simulink model "ES101A_DiagcMgr"  (R2013b)
settings: Solver=ode45  StartTime=0.0  StopTime=0.44  RelTol=1e-3
values from neighbouring files (symbols this model uses):
  BrdgVltg = DataDict.IpSignal    [ES101A_DiagcMgr_DataDict.m]
  DEM_CLEAR_PENDING = DataDict.Constant    [ES101A_DiagcMgr_DataDict.m]
  DEM_DTC_GROUP_ALL_DTCS = DataDict.Constant    [ES101A_DiagcMgr_DataDict.m]
  DFTAGICNTR_CNT_U08 = DataDict.Constant    [ES101A_DiagcMgr_DataDict.m]
  DIAGCMGR_NTCINFOSTSTESTFAILD_CNT_U08 = DataDict.Constant    [ES101A_DiagcMgr_DataDict.m]
  DIAGCMGR_NTCINFOSTSTESTFAILDTHISIGNCYC_CNT_U08 = DataDict.Constant    [ES101A_DiagcMgr_DataDict.m]
  DIAGCMGR_NTCINFOSTSTESTNOTCMPLTHISIGNCYC_CNT_U08 = DataDict.Constant    [ES101A_DiagcMgr_DataDict.m]
  DiagcMgrFltResp = DataDict.Calibration    [ES101A_DiagcMgr_DataDict.m]
  DiagcMgrNtcFltAry = DataDict.NVM    [ES101A_DiagcMgr_DataDict.m]
  DIAGCSTSCTRLDSHTDWNFLTPRSNT_CNT_U16 = DataDict.Constant    [ES101A_DiagcMgr_DataDict.m]
  DIAGCSTSDFTHWAG_CNT_U16 = DataDict.Constant    [ES101A_DiagcMgr_DataDict.m]
  DIAGCSTSDFTHWAGSERLCOMEXPRTVAL_CNT_U16 = DataDict.Constant    [ES101A_DiagcMgr_DataDict.m]
  DIAGCSTSDFTVEHSPD_CNT_U16 = DataDict.Constant    [ES101A_DiagcMgr_DataDict.m]
  DIAGCSTSININVAL_CNT_U16 = DataDict.Constant    [ES101A_DiagcMgr_DataDict.m]
  DIAGCSTSIVTR1INACTV_CNT_U16 = DataDict.Constant    [ES101A_DiagcMgr_DataDict.m]
  DIAGCSTSIVTR2INACTV_CNT_U16 = DataDict.Constant    [ES101A_DiagcMgr_DataDict.m]
  DIAGCSTSLIMDTPRFMNC_CNT_U16 = DataDict.Constant    [ES101A_DiagcMgr_DataDict.m]
  DIAGCSTSRAMPTOZEROFLTPRSNT_CNT_U16 = DataDict.Constant    [ES101A_DiagcMgr_DataDict.m]
  DIAGCSTSWHLIMBREJCTNDI_CNT_U16 = DataDict.Constant    [ES101A_DiagcMgr_DataDict.m]
  DTCIDXSTSFAIL_CNT_U08 = DataDict.Constant    [ES101A_DiagcMgr_DataDict.m]
  DTCIDXSTSNONTC_CNT_U08 = DataDict.Constant    [ES101A_DiagcMgr_DataDict.m]
  DTCIDXSTSNORES_CNT_U08 = DataDict.Constant    [ES101A_DiagcMgr_DataDict.m]
  DTCIDXSTSPASS_CNT_U08 = DataDict.Constant    [ES101A_DiagcMgr_DataDict.m]
  DTCIDXSTSUPDCFMD_CNT_U08 = DataDict.Constant    [ES101A_DiagcMgr_DataDict.m]
  ELECGLBPRM_IVTRCNT_CNT_U08 = DataDict.ConfigParam    [ES101A_DiagcMgr_DataDict.m]
  FLTINJ_DIAGCMGR_DIAGCSTSIVTR1INACTV = DataDict.Constant    [ES101A_DiagcMgr_DataDict.m]
  FLTINJ_DIAGCMGR_DIAGCSTSIVTR2INACTV = DataDict.Constant    [ES101A_DiagcMgr_DataDict.m]
  HwTq = DataDict.IpSignal    [ES101A_DiagcMgr_DataDict.m]
  IgnCntr = DataDict.IpSignal    [ES101A_DiagcMgr_DataDict.m]
  MAXDEBCNTRVAL_CNT_S16 = DataDict.Constant    [ES101A_DiagcMgr_DataDict.m]
  MAXRAMPRATE_ULSPERSEC_F32 = DataDict.Constant    [ES101A_DiagcMgr_DataDict.m]
  MINDEBCNTRVAL_CNT_S16 = DataDict.Constant    [ES101A_DiagcMgr_DataDict.m]
  MINRAMPRATE_ULSPERSEC_F32 = DataDict.Constant    [ES101A_DiagcMgr_DataDict.m]
  SCAMOTTQCMDTOONE_ULS_F32 = DataDict.Constant    [ES101A_DiagcMgr_DataDict.m]
  SCAMOTTQCMDTOZERO_ULS_F32 = DataDict.Constant    [ES101A_DiagcMgr_DataDict.m]
  SysSt = DataDict.IpSignal    [ES101A_DiagcMgr_DataDict.m]
  VehSpd = DataDict.IpSignal    [ES101A_DiagcMgr_DataDict.m]
undefined symbols (not defined in the file or in its folder): ActvMotTqCmdSca, ActvRampRate, AgiCntr, Dem_DTCFormatType, Dem_DTCOriginType, Dem_EventStatusType, DiagcData, DiagcMgrNtcMap, DiagcSts, DtcEnaMask, EcuT, HistNtcFltAry, MicroDiagcData, MotTq, NtcNr, NtcNrWithResd1, NtcStInfo, ProxySetNtcData, Sts, SysSt1, TOTNROFDTC_CNT_U08
libraries: simulink x151, FloatToFixd x5, NxtrNvM x4
(part 5 of 13)

== system ES101A_DiagcMgr/DiagcMgr/DiagcMgrPer2/Normal Periodic Processing/For All DTCs ==
  CopyRight2 : Subsystem  Description=|  mask(Copyright Information){none=on}
      | Copyright info block.                                               
      |                                                                     
      | Place copyright information at the top of every subsystem in design.
      mask prompts: none "No parameters"
      mask help: Place copyright information at the top of every subsystem in design.
      mask Display:
      | NxtrConf = 'Nexteer Confidential';
      | 
      | sys = bdroot; %handle for the current model ("system")
      | first = get_param(sys,'Created');
      | first = first(end-3:end);  %year is last four digits
      | 
      | last = get_param(sys,'LastModifiedDate');
      | if isempty(last)
      |     last = datestr(now,'yyyy');
      | else
      |     last = last(end-3:end);
      | end
      | 
      | if strcmp(first,last)
      |     fprintf('%s -- Copyright %s Nexteer',NxtrConf,first)
      | else
      |     fprintf('%s -- %s%s- %s Nexteer',NxtrConf,char(169),first,last)
      | end
  Data Store Read1 : DataStoreRead  DataStoreName=DtcIdxCurrSts
  Data Store Read2 : DataStoreRead  DataStoreName=DtcIdxPrevSts
  For Each DTC : Subsystem  TreatAsAtomicUnit=on
  For Iterator : ForIterator  IterationLimit=TOTNROFDTC_CNT_U08 + 1  IndexMode=Zero-based
  Selector1 : Selector  IndexMode=Zero-based  InputPortWidth=512  IndexOptions=Index vector (port)  Indices=[1 3]  OutputSizes=1
  Selector2 : Selector  IndexMode=Zero-based  InputPortWidth=512  IndexOptions=Index vector (port)  Indices=[1 3]  OutputSizes=1
  wires:
  For Iterator/1 -> Selector1/2, For Each DTC/2(DtcIdx), Selector2/2
  Data Store Read2/1 -> Selector1/1
  Selector1/1 -> For Each DTC/3(DtcIdxPrevSts)
  Data Store Read1/1 -> Selector2/1
  Selector2/1 -> For Each DTC/1(DtcIdxCurrSts)

== system ES101A_DiagcMgr/DiagcMgr/DiagcMgrPer2/Normal Periodic Processing/For All NTCs ==
  Bus Selector1 : BusSelector  OutputSignals=ApplIdx,NtcInfoIdx
  CopyRight2 : Subsystem  Description=|  mask(Copyright Information){none=on}
      | Copyright info block.                                               
      |                                                                     
      | Place copyright information at the top of every subsystem in design.
      mask prompts: none "No parameters"
      mask help: Place copyright information at the top of every subsystem in design.
      mask Display:
      | NxtrConf = 'Nexteer Confidential';
      | 
      | sys = bdroot; %handle for the current model ("system")
      | first = get_param(sys,'Created');
      | first = first(end-3:end);  %year is last four digits
      | 
      | last = get_param(sys,'LastModifiedDate');
      | if isempty(last)
      |     last = datestr(now,'yyyy');
      | else
      |     last = last(end-3:end);
      | end
      | 
      | if strcmp(first,last)
      |     fprintf('%s -- Copyright %s Nexteer',NxtrConf,first)
      | else
      |     fprintf('%s -- %s%s- %s Nexteer',NxtrConf,char(169),first,last)
      | end
  Data Store Read2 : DataStoreRead  DataStoreName=DiagcMgrNtcMap  DataStoreElements=DiagcMgrNtcMap(:)
  For Each NTC : Subsystem  TreatAsAtomicUnit=on
  For Iterator : ForIterator  IterationLimit=511
  Selector1 : Selector  IndexMode=Zero-based  InputPortWidth=512  IndexOptions=Index vector (port)  Indices=[1 3]  OutputSizes=1
  wires:
  Data Store Read2/1 -> Selector1/1
  Selector1/1 -> Bus Selector1/1
  Bus Selector1/1 -> For Each NTC/1(ApplIdx)  "<ApplIdx>"
  Bus Selector1/2 -> For Each NTC/2(NtcInfoIdx)  "<NtcInfoIdx>"
  For Iterator/1 -> For Each NTC/3(NtcNr), Selector1/2

== system ES101A_DiagcMgr/DiagcMgr/DiagcMgrPer2/Normal Periodic Processing/Initialize DtcIdxCurrSts ==
  Assignment : Assignment  IndexMode=Zero-based  IndexOptions=Starting index (port)  Indices=1  OutputSizes=1
  CopyRight2 : Subsystem  Description=|  mask(Copyright Information){none=on}
      | Copyright info block.                                               
      |                                                                     
      | Place copyright information at the top of every subsystem in design.
      mask prompts: none "No parameters"
      mask help: Place copyright information at the top of every subsystem in design.
      mask Display:
      | NxtrConf = 'Nexteer Confidential';
      | 
      | sys = bdroot; %handle for the current model ("system")
      | first = get_param(sys,'Created');
      | first = first(end-3:end);  %year is last four digits
      | 
      | last = get_param(sys,'LastModifiedDate');
      | if isempty(last)
      |     last = datestr(now,'yyyy');
      | else
      |     last = last(end-3:end);
      | end
      | 
      | if strcmp(first,last)
      |     fprintf('%s -- Copyright %s Nexteer',NxtrConf,first)
      | else
      |     fprintf('%s -- %s%s- %s Nexteer',NxtrConf,char(169),first,last)
      | end
  Data Store Read : DataStoreRead  DataStoreName=DtcIdxCurrSts
  Data Store Write : DataStoreWrite  DataStoreName=DtcIdxCurrSts
  For Iterator : ForIterator  IterationLimit=TOTNROFDTC_CNT_U08+1  IndexMode=Zero-based
  No NTC : Constant  Value=DTCIDXSTSNONTC_CNT_U08
  wires:
  For Iterator/1 -> Assignment/3
  Assignment/1 -> Data Store Write/1
  No NTC/1 -> Assignment/2
  Data Store Read/1 -> Assignment/1

== system ES101A_DiagcMgr/DiagcMgr/DiagcMgrPwrDwn/Clear NtcFltAryIdx and HistFltAryIdx/CopyRight2 ==

== system ES101A_DiagcMgr/DiagcMgr/DiagcMgrPwrDwn/Update NtcFltAry and HistFltAry/CopyRight2 ==

== system ES101A_DiagcMgr/DiagcMgr/DiagcMgrPwrDwn/Update NtcFltAry and HistFltAry/For Number of NTCs ==
  note: SW Implementation:
      |
      | 	SW uses a switched case with ApplIdx as the input. The GetNtcInfoApplX is
      | 	called inside each of the switched case statements. Based on the application
      | 	index, the respective NtcInfoAryX is selected.
  ApplIdx : Inport
  NtcInfoIdx : Inport  Port=2
  NtcMapIdx : Inport  Port=3
  Bus Selector1 : BusSelector  OutputSignals=AgiCntr,Sts
  Check Aging Counter : Subsystem  TreatAsAtomicUnit=on
  CopyRight2 : Subsystem  Description=|  mask(Copyright Information){none=on}
      | Copyright info block.                                               
      |                                                                     
      | Place copyright information at the top of every subsystem in design.
      mask prompts: none "No parameters"
      mask help: Place copyright information at the top of every subsystem in design.
      mask Display:
      | NxtrConf = 'Nexteer Confidential';
      | 
      | sys = bdroot; %handle for the current model ("system")
      | first = get_param(sys,'Created');
      | first = first(end-3:end);  %year is last four digits
      | 
      | last = get_param(sys,'LastModifiedDate');
      | if isempty(last)
      |     last = datestr(now,'yyyy');
      | else
      |     last = last(end-3:end);
      | end
      | 
      | if strcmp(first,last)
      |     fprintf('%s -- Copyright %s Nexteer',NxtrConf,first)
      | else
      |     fprintf('%s -- %s%s- %s Nexteer',NxtrConf,char(169),first,last)
      | end
  Default Case : Subsystem  TreatAsAtomicUnit=on
  GetNtcInfoAppIX : Subsystem  TreatAsAtomicUnit=on
  Merge : Merge
  Merge1 : Merge
  Switch Case : SwitchCase  CaseConditions={X}
  wires:
  NtcMapIdx/1 -> Check Aging Counter/1(NtcMapIdx)
  ApplIdx/1 -> Switch Case/1
  NtcInfoIdx/1 -> GetNtcInfoAppIX/1(NtcInfoIdx_ArgIn)
  Switch Case/1 -> GetNtcInfoAppIX/Action
  Switch Case/2 -> Default Case/Action
  GetNtcInfoAppIX/1(NtcInfo_ArgOut) -> Bus Selector1/1
  Bus Selector1/1 -> Merge/1  "<AgiCntr>"
  Default Case/1(AgiCntr) -> Merge/2
  Merge/1 -> Check Aging Counter/2(AgiCntr)
  Merge1/1 -> Check Aging Counter/3(Sts)
  Bus Selector1/2 -> Merge1/1  "<Sts>"
  Default Case/2(Sts) -> Merge1/2

== system ES101A_DiagcMgr/DiagcMgr/DiagcMgrPwrDwn/While((HistFltAryTempIdx < HistFltInfoIdx) AND (NtcFltAryIdx < 20))/CopyRight1 ==

== system ES101A_DiagcMgr/DiagcMgr/DiagcMgrPwrDwn/While((HistFltAryTempIdx < HistFltInfoIdx) AND (NtcFltAryIdx < 20))/Increment HistFltAryTempIdx and NtcFltAryIdx ==
  Add : Sum
  Add1 : Sum
  Constant : Constant  OutDataTypeStr=uint8
  Constant1 : Constant  OutDataTypeStr=uint8
  CopyRight1 : Subsystem  Description=|  mask(Copyright Information){none=on}
      | Copyright info block.                                               
      |                                                                     
      | Place copyright information at the top of every subsystem in design.
      mask prompts: none "No parameters"
      mask help: Place copyright information at the top of every subsystem in design.
      mask Display:
      | NxtrConf = 'Nexteer Confidential';
      | 
      | sys = bdroot; %handle for the current model ("system")
      | first = get_param(sys,'Created');
      | first = first(end-3:end);  %year is last four digits
      | 
      | last = get_param(sys,'LastModifiedDate');
      | if isempty(last)
      |     last = datestr(now,'yyyy');
      | else
      |     last = last(end-3:end);
      | end
      | 
      | if strcmp(first,last)
      |     fprintf('%s -- Copyright %s Nexteer',NxtrConf,first)
      | else
      |     fprintf('%s -- %s%s- %s Nexteer',NxtrConf,char(169),first,last)
      | end
  Data Store Read1 : DataStoreRead  DataStoreName=NtcFltAryIdx
  Data Store Read4 : DataStoreRead  DataStoreName=HistFltAryTempIdx
  Data Store Write1 : DataStoreWrite  DataStoreName=HistFltAryTempIdx
  Data Store Write2 : DataStoreWrite  DataStoreName=NtcFltAryIdx
  wires:
  Add/1 -> Data Store Write1/1
  Constant/1 -> Add/2
  Data Store Read4/1 -> Add/1
  Add1/1 -> Data Store Write2/1
  Constant1/1 -> Add1/2
  Data Store Read1/1 -> Add1/1

== system ES101A_DiagcMgr/DiagcMgr/DiagcMgrPwrDwn/While((HistFltAryTempIdx < HistFltInfoIdx) AND (NtcFltAryIdx < 20))/Update NtcFltAry ==
  Assignment1 : Assignment  IndexMode=Zero-based  IndexOptions=Index vector (port)  Indices=1  OutputSizes=1
  CopyRight1 : Subsystem  Description=|  mask(Copyright Information){none=on}
      | Copyright info block.                                               
      |                                                                     
      | Place copyright information at the top of every subsystem in design.
      mask prompts: none "No parameters"
      mask help: Place copyright information at the top of every subsystem in design.
      mask Display:
      | NxtrConf = 'Nexteer Confidential';
      | 
      | sys = bdroot; %handle for the current model ("system")
      | first = get_param(sys,'Created');
      | first = first(end-3:end);  %year is last four digits
      | 
      | last = get_param(sys,'LastModifiedDate');
      | if isempty(last)
      |     last = datestr(now,'yyyy');
      | else
      |     last = last(end-3:end);
      | end
      | 
      | if strcmp(first,last)
      |     fprintf('%s -- Copyright %s Nexteer',NxtrConf,first)
      | else
      |     fprintf('%s -- %s%s- %s Nexteer',NxtrConf,char(169),first,last)
      | end
  Data Store Write2 : DataStoreWrite  DataStoreName=DiagcMgrNtcFltAry  DataStoreElements=DiagcMgrNtcFltAry(:)
  Data Store Read1 : DataStoreRead  DataStoreName=HistNtcFltAry
  Data Store Read2 : DataStoreRead  DataStoreName=NtcFltAryIdx
  Data Store Read3 : DataStoreRead  DataStoreName=HistFltAryTempIdx
  Data Store Read4 : DataStoreRead  DataStoreName=DiagcMgrNtcFltAry
  Selector1 : Selector  IndexMode=Zero-based  InputPortWidth=20  IndexOptions=Index vector (port)  Indices=[1 3]  OutputSizes=1
  wires:
  Data Store Read1/1 -> Selector1/1
  Data Store Read3/1 -> Selector1/2
  Selector1/1 -> Assignment1/2
  Assignment1/1 -> Data Store Write2/1
  Data Store Read2/1 -> Assignment1/3
  Data Store Read4/1 -> Assignment1/1

== system ES101A_DiagcMgr/DiagcMgr/DiagcMgrPwrDwn/While(CurrentFltIdx < TableSize[NtcFltAry])/CopyRight1 ==

== system ES101A_DiagcMgr/DiagcMgr/DiagcMgrPwrDwn/While(CurrentFltIdx < TableSize[NtcFltAry])/Increment Indices ==
  Add1 : Sum
  Constant1 : Constant  OutDataTypeStr=uint8
  CopyRight1 : Subsystem  Description=|  mask(Copyright Information){none=on}
      | Copyright info block.                                               
      |                                                                     
      | Place copyright information at the top of every subsystem in design.
      mask prompts: none "No parameters"
      mask help: Place copyright information at the top of every subsystem in design.
      mask Display:
      | NxtrConf = 'Nexteer Confidential';
      | 
      | sys = bdroot; %handle for the current model ("system")
      | first = get_param(sys,'Created');
      | first = first(end-3:end);  %year is last four digits
      | 
      | last = get_param(sys,'LastModifiedDate');
      | if isempty(last)
      |     last = datestr(now,'yyyy');
      | else
      |     last = last(end-3:end);
      | end
      | 
      | if strcmp(first,last)
      |     fprintf('%s -- Copyright %s Nexteer',NxtrConf,first)
      | else
      |     fprintf('%s -- %s%s- %s Nexteer',NxtrConf,char(169),first,last)
      | end
  Data Store Read6 : DataStoreRead  DataStoreName=NtcFltAryIdx
  Data Store Write3 : DataStoreWrite  DataStoreName=NtcFltAryIdx
  wires:
  Data Store Read6/1 -> Add1/1
  Constant1/1 -> Add1/2
  Add1/1 -> Data Store Write3/1

== system ES101A_DiagcMgr/DiagcMgr/DiagcMgrPwrDwn/While(CurrentFltIdx < TableSize[NtcFltAry])/Update NtcFltAry ==
  Assignment1 : Assignment  IndexMode=Zero-based  IndexOptions=Index vector (port)  Indices=1  OutputSizes=1
  Bus Assignment1 : BusAssignment  AssignedSignals=NtcNr,AgiCntr,Sts
  Constant : Constant  Value=0  OutDataTypeStr=uint16
  Constant1 : Constant  Value=DFTAGICNTR_CNT_U08
  Constant2 : Constant  Value=0  OutDataTypeStr=uint8
  CopyRight1 : Subsystem  Description=|  mask(Copyright Information){none=on}
      | Copyright info block.                                               
      |                                                                     
      | Place copyright information at the top of every subsystem in design.
      mask prompts: none "No parameters"
      mask help: Place copyright information at the top of every subsystem in design.
      mask Display:
      | NxtrConf = 'Nexteer Confidential';
      | 
      | sys = bdroot; %handle for the current model ("system")
      | first = get_param(sys,'Created');
      | first = first(end-3:end);  %year is last four digits
      | 
      | last = get_param(sys,'LastModifiedDate');
      | if isempty(last)
      |     last = datestr(now,'yyyy');
      | else
      |     last = last(end-3:end);
      | end
      | 
      | if strcmp(first,last)
      |     fprintf('%s -- Copyright %s Nexteer',NxtrConf,first)
      | else
      |     fprintf('%s -- %s%s- %s Nexteer',NxtrConf,char(169),first,last)
      | end
  Data Store Write2 : DataStoreWrite  DataStoreName=DiagcMgrNtcFltAry  DataStoreElements=DiagcMgrNtcFltAry(:)
  Data Store Read1 : DataStoreRead  DataStoreName=DiagcMgrNtcFltAry
  Data Store Read3 : DataStoreRead  DataStoreName=NtcFltAryIdx
  Selector1 : Selector  IndexMode=Zero-based  InputPortWidth=20  IndexOptions=Index vector (port)  Indices=[1 3]  OutputSizes=1
  wires:
  Selector1/1 -> Bus Assignment1/1
  Data Store Read1/1 -> Selector1/1, Assignment1/1
  Data Store Read3/1 -> Selector1/2, Assignment1/3
  Bus Assignment1/1 -> Assignment1/2
  Assignment1/1 -> Data Store Write2/1
  Constant/1 -> Bus Assignment1/2
  Constant1/1 -> Bus Assignment1/3
  Constant2/1 -> Bus Assignment1/4

== system ES101A_DiagcMgr/DiagcMgr/DiagcMgrPwrDwn/Write to NvM/CopyRight2 ==

== system ES101A_DiagcMgr/DiagcMgr/GetNtcActvCore /GetNtcInfoAppIX/CopyRight2 ==

== system ES101A_DiagcMgr/DiagcMgr/GetNtcActvCore /NTC Not Active/CopyRight2 ==

== system ES101A_DiagcMgr/DiagcMgr/GetNtcQlfrStsCore /GetNtcInfoAppIX/CopyRight2 ==

== system ES101A_DiagcMgr/DiagcMgr/GetNtcQlfrStsCore /No Result State/CopyRight2 ==

== system ES101A_DiagcMgr/DiagcMgr/GetNtcStsCore/GetNtcInfoAppIX/CopyRight2 ==

== system ES101A_DiagcMgr/DiagcMgr/GetNtcStsCore/NTC Default Status/CopyRight2 ==

== system ES101A_DiagcMgr/DiagcMgr/ReadNtcFltAry/Initialize NtcMapIdx Clear HistReadFltAryIdx, ReadFltAryIdx and HistReadFltAryTempIdx/CopyRight2 ==

== system ES101A_DiagcMgr/DiagcMgr/ReadNtcFltAry/Send out data/CopyRight2 ==

== system ES101A_DiagcMgr/DiagcMgr/ReadNtcFltAry/Update DiagcMgrReadFltInfoAry and HistReadFltAry/CopyRight2 ==

== system ES101A_DiagcMgr/DiagcMgr/ReadNtcFltAry/Update DiagcMgrReadFltInfoAry and HistReadFltAry/For Number of NTCs ==
  note: SW Implementation:
      |
      | 	SW uses a switched case with ApplIdx as the input. The GetNtcInfoApplX is
      | 	called inside each of the switched case statements. Based on the application
      | 	index, the respective NtcInfoAryX is selected.
  ApplIdx : Inport
  NtcInfoIdx : Inport  Port=2
  NtcMapIdx : Inport  Port=3
  Bus Selector2 : BusSelector  OutputSignals=AgiCntr,Sts,NtcStInfo
  Check Aging Counter : Subsystem  TreatAsAtomicUnit=on
  CopyRight2 : Subsystem  Description=|  mask(Copyright Information){none=on}
      | Copyright info block.                                               
      |                                                                     
      | Place copyright information at the top of every subsystem in design.
      mask prompts: none "No parameters"
      mask help: Place copyright information at the top of every subsystem in design.
      mask Display:
      | NxtrConf = 'Nexteer Confidential';
      | 
      | sys = bdroot; %handle for the current model ("system")
      | first = get_param(sys,'Created');
      | first = first(end-3:end);  %year is last four digits
      | 
      | last = get_param(sys,'LastModifiedDate');
      | if isempty(last)
      |     last = datestr(now,'yyyy');
      | else
      |     last = last(end-3:end);
      | end
      | 
      | if strcmp(first,last)
      |     fprintf('%s -- Copyright %s Nexteer',NxtrConf,first)
      | else
      |     fprintf('%s -- %s%s- %s Nexteer',NxtrConf,char(169),first,last)
      | end
  Default Case : Subsystem  TreatAsAtomicUnit=on
  GetNtcInfoAppIX : Subsystem  TreatAsAtomicUnit=on
  Merge : Merge
  Merge1 : Merge
  Merge2 : Merge
  Switch Case : SwitchCase  CaseConditions={X}
  wires:
  NtcMapIdx/1 -> Check Aging Counter/1(NtcMapIdx)
  NtcInfoIdx/1 -> GetNtcInfoAppIX/1(NtcInfoIdx_ArgIn)
  Switch Case/1 -> GetNtcInfoAppIX/Action
  Switch Case/2 -> Default Case/Action
  ApplIdx/1 -> Switch Case/1
  GetNtcInfoAppIX/1(NtcInfo_ArgOut) -> Bus Selector2/1
  Bus Selector2/1 -> Merge/1  "<AgiCntr>"
  Default Case/1(AgiCntr) -> Merge/2
  Bus Selector2/2 -> Merge1/1  "<Sts>"
  Default Case/2(Sts) -> Merge1/2
  Bus Selector2/3 -> Merge2/1  "<NtcStInfo>"
  Default Case/3(NtcStInfo) -> Merge2/2
  Merge2/1 -> Check Aging Counter/4(NtcStInfo)
  Merge1/1 -> Check Aging Counter/3(Sts)
  Merge/1 -> Check Aging Counter/2(AgiCntr)

== system ES101A_DiagcMgr/DiagcMgr/ReadNtcFltAry/While((HistReadFltAryTempIdx < HistReadFltAryIdx) AND (ReadFltInfoIndx < 20))/CopyRight1 ==

== system ES101A_DiagcMgr/DiagcMgr/ReadNtcFltAry/While((HistReadFltAryTempIdx < HistReadFltAryIdx) AND (ReadFltInfoIndx < 20))/Increment HistFltAryTempdx and NtcFltAryIdx ==
  Add : Sum
  Add1 : Sum
  Constant : Constant  OutDataTypeStr=uint8
  Constant1 : Constant  OutDataTypeStr=uint8
  CopyRight1 : Subsystem  Description=|  mask(Copyright Information){none=on}
      | Copyright info block.                                               
      |                                                                     
      | Place copyright information at the top of every subsystem in design.
      mask prompts: none "No parameters"
      mask help: Place copyright information at the top of every subsystem in design.
      mask Display:
      | NxtrConf = 'Nexteer Confidential';
      | 
      | sys = bdroot; %handle for the current model ("system")
      | first = get_param(sys,'Created');
      | first = first(end-3:end);  %year is last four digits
      | 
      | last = get_param(sys,'LastModifiedDate');
      | if isempty(last)
      |     last = datestr(now,'yyyy');
      | else
      |     last = last(end-3:end);
      | end
      | 
      | if strcmp(first,last)
      |     fprintf('%s -- Copyright %s Nexteer',NxtrConf,first)
      | else
      |     fprintf('%s -- %s%s- %s Nexteer',NxtrConf,char(169),first,last)
      | end
  Data Store Read1 : DataStoreRead  DataStoreName=ReadFltInfoIdx
  Data Store Read4 : DataStoreRead  DataStoreName=HistFltAryTempIdx
  Data Store Write1 : DataStoreWrite  DataStoreName=HistFltAryTempIdx
  Data Store Write2 : DataStoreWrite  DataStoreName=ReadFltInfoIdx
  wires:
  Add/1 -> Data Store Write1/1
  Constant/1 -> Add/2
  Data Store Read4/1 -> Add/1
  Add1/1 -> Data Store Write2/1
  Constant1/1 -> Add1/2
  Data Store Read1/1 -> Add1/1

== system ES101A_DiagcMgr/DiagcMgr/ReadNtcFltAry/While((HistReadFltAryTempIdx < HistReadFltAryIdx) AND (ReadFltInfoIndx < 20))/Update NtcFltAry ==
  Assignment1 : Assignment  IndexMode=Zero-based  IndexOptions=Index vector (port)  Indices=1  OutputSizes=1
  CopyRight1 : Subsystem  Description=|  mask(Copyright Information){none=on}
      | Copyright info block.                                               
      |                                                                     
      | Place copyright information at the top of every subsystem in design.
      mask prompts: none "No parameters"
      mask help: Place copyright information at the top of every subsystem in design.
      mask Display:
      | NxtrConf = 'Nexteer Confidential';
      | 
      | sys = bdroot; %handle for the current model ("system")
      | first = get_param(sys,'Created');
      | first = first(end-3:end);  %year is last four digits
      | 
      | last = get_param(sys,'LastModifiedDate');
      | if isempty(last)
      |     last = datestr(now,'yyyy');
      | else
      |     last = last(end-3:end);
      | end
      | 
      | if strcmp(first,last)
      |     fprintf('%s -- Copyright %s Nexteer',NxtrConf,first)
      | else
      |     fprintf('%s -- %s%s- %s Nexteer',NxtrConf,char(169),first,last)
      | end
  Data Store Write2 : DataStoreWrite  DataStoreName=DiagcMgrReadFltInfoAry
  Data Store Read1 : DataStoreRead  DataStoreName=HistReadFltAry
  Data Store Read2 : DataStoreRead  DataStoreName=ReadFltInfoIdx
  Data Store Read3 : DataStoreRead  DataStoreName=HistReadFltAryTempIdx
  Data Store Read4 : DataStoreRead  DataStoreName=DiagcMgrReadFltInfoAry
  Selector1 : Selector  IndexMode=Zero-based  InputPortWidth=20  IndexOptions=Index vector (port)  Indices=[1 3]  OutputSizes=1
  wires:
  Data Store Read1/1 -> Selector1/1
  Data Store Read3/1 -> Selector1/2
  Selector1/1 -> Assignment1/2
  Assignment1/1 -> Data Store Write2/1
  Data Store Read2/1 -> Assignment1/3
  Data Store Read4/1 -> Assignment1/1

== system ES101A_DiagcMgr/DiagcMgr/ReadNtcFltAry/While(ReadFltInfoIdx < TableSize[DiagcMgrReadFltInfoAry])/CopyRight1 ==

== system ES101A_DiagcMgr/DiagcMgr/ReadNtcFltAry/While(ReadFltInfoIdx < TableSize[DiagcMgrReadFltInfoAry])/Increment Indices ==
  Add1 : Sum
  Constant1 : Constant  OutDataTypeStr=uint8
  CopyRight1 : Subsystem  Description=|  mask(Copyright Information){none=on}
      | Copyright info block.                                               
      |                                                                     
      | Place copyright information at the top of every subsystem in design.
      mask prompts: none "No parameters"
      mask help: Place copyright information at the top of every subsystem in design.
      mask Display:
      | NxtrConf = 'Nexteer Confidential';
      | 
      | sys = bdroot; %handle for the current model ("system")
      | first = get_param(sys,'Created');
      | first = first(end-3:end);  %year is last four digits
      | 
      | last = get_param(sys,'LastModifiedDate');
      | if isempty(last)
      |     last = datestr(now,'yyyy');
      | else
      |     last = last(end-3:end);
      | end
      | 
      | if strcmp(first,last)
      |     fprintf('%s -- Copyright %s Nexteer',NxtrConf,first)
      | else
      |     fprintf('%s -- %s%s- %s Nexteer',NxtrConf,char(169),first,last)
      | end
  Data Store Read6 : DataStoreRead  DataStoreName=ReadFltInfoIdx
  Data Store Write3 : DataStoreWrite  DataStoreName=ReadFltInfoIdx
  wires:
  Data Store Read6/1 -> Add1/1
  Constant1/1 -> Add1/2
  Add1/1 -> Data Store Write3/1

== system ES101A_DiagcMgr/DiagcMgr/ReadNtcFltAry/While(ReadFltInfoIdx < TableSize[DiagcMgrReadFltInfoAry])/Update NtcFltAry ==
  Assignment1 : Assignment  IndexMode=Zero-based  IndexOptions=Index vector (port)  Indices=1  OutputSizes=1
  Bus Assignment1 : BusAssignment  AssignedSignals=NtcNr,AgiCntr,Sts
  Constant : Constant  Value=0  OutDataTypeStr=uint16
  Constant1 : Constant  Value=DFTAGICNTR_CNT_U08
  Constant2 : Constant  Value=0  OutDataTypeStr=uint8
  CopyRight1 : Subsystem  Description=|  mask(Copyright Information){none=on}
      | Copyright info block.                                               
      |                                                                     
      | Place copyright information at the top of every subsystem in design.
      mask prompts: none "No parameters"
      mask help: Place copyright information at the top of every subsystem in design.
      mask Display:
      | NxtrConf = 'Nexteer Confidential';
      | 
      | sys = bdroot; %handle for the current model ("system")
      | first = get_param(sys,'Created');
      | first = first(end-3:end);  %year is last four digits
      | 
      | last = get_param(sys,'LastModifiedDate');
      | if isempty(last)
      |     last = datestr(now,'yyyy');
      | else
      |     last = last(end-3:end);
      | end
      | 
      | if strcmp(first,last)
      |     fprintf('%s -- Copyright %s Nexteer',NxtrConf,first)
      | else
      |     fprintf('%s -- %s%s- %s Nexteer',NxtrConf,char(169),first,last)
      | end
  Data Store Write2 : DataStoreWrite  DataStoreName=DiagcMgrReadFltInfoAry
  Data Store Read1 : DataStoreRead  DataStoreName=DiagcMgrReadFltInfoAry
  Data Store Read3 : DataStoreRead  DataStoreName=ReadFltInfoIdx
  Selector1 : Selector  IndexMode=Zero-based  InputPortWidth=20  IndexOptions=Index vector (port)  Indices=[1 3]  OutputSizes=1
  wires:
  Selector1/1 -> Bus Assignment1/1
  Data Store Read1/1 -> Selector1/1, Assignment1/1
  Data Store Read3/1 -> Selector1/2, Assignment1/3
  Bus Assignment1/1 -> Assignment1/2
  Assignment1/1 -> Data Store Write2/1
  Constant/1 -> Bus Assignment1/2
  Constant1/1 -> Bus Assignment1/3
  Constant2/1 -> Bus Assignment1/4

== system ES101A_DiagcMgr/DiagcMgr/ReadNtcInfoAndDebCntr/ApplX/CopyRight2 ==

== system ES101A_DiagcMgr/DiagcMgr/ReadNtcInfoAndDebCntr/ApplX/Debounced ==
  DebCntrIdx_ArgIn : Inport
  Action Port : ActionPort  ActionType=else
  CopyRight2 : Subsystem  Description=|  mask(Copyright Information){none=on}
      | Copyright info block.                                               
      |                                                                     
      | Place copyright information at the top of every subsystem in design.
      mask prompts: none "No parameters"
      mask help: Place copyright information at the top of every subsystem in design.
      mask Display:
      | NxtrConf = 'Nexteer Confidential';
      | 
      | sys = bdroot; %handle for the current model ("system")
      | first = get_param(sys,'Created');
      | first = first(end-3:end);  %year is last four digits
      | 
      | last = get_param(sys,'LastModifiedDate');
      | if isempty(last)
      |     last = datestr(now,'yyyy');
      | else
      |     last = last(end-3:end);
      | end
      | 
      | if strcmp(first,last)
      |     fprintf('%s -- Copyright %s Nexteer',NxtrConf,first)
      | else
      |     fprintf('%s -- %s%s- %s Nexteer',NxtrConf,char(169),first,last)
      | end
  GetNtcDebCntrApplX : Subsystem  TreatAsAtomicUnit=on
  DebCntr_ArgOut : Outport
  wires:
  GetNtcDebCntrApplX/1(DebCntr_ArgOut) -> DebCntr_ArgOut/1
  DebCntrIdx_ArgIn/1 -> GetNtcDebCntrApplX/1(DebCntrIdx_ArgIn)

== system ES101A_DiagcMgr/DiagcMgr/ReadNtcInfoAndDebCntr/ApplX/GetNtcInfoAppIX ==
  NtcInfoIdx_ArgIn : Inport
  CopyRight2 : Subsystem  Description=|  mask(Copyright Information){none=on}
      | Copyright info block.                                               
      |                                                                     
      | Place copyright information at the top of every subsystem in design.
      mask prompts: none "No parameters"
      mask help: Place copyright information at the top of every subsystem in design.
      mask Display:
      | NxtrConf = 'Nexteer Confidential';
      | 
      | sys = bdroot; %handle for the current model ("system")
      | first = get_param(sys,'Created');
      | first = first(end-3:end);  %year is last four digits
      | 
      | last = get_param(sys,'LastModifiedDate');
      | if isempty(last)
      |     last = datestr(now,'yyyy');
      | else
      |     last = last(end-3:end);
      | end
      | 
      | if strcmp(first,last)
      |     fprintf('%s -- Copyright %s Nexteer',NxtrConf,first)
      | else
      |     fprintf('%s -- %s%s- %s Nexteer',NxtrConf,char(169),first,last)
      | end
  Data Store Read : DataStoreRead  DataStoreName=DiagcMgrNtcInfoX
  Selector : Selector  IndexMode=Zero-based  InputPortWidth=14  IndexOptions=Index vector (port)  Indices=[1 3]  OutputSizes=1
  NtcInfo_ArgOut : Outport
  wires:
  Selector/1 -> NtcInfo_ArgOut/1
  NtcInfoIdx_ArgIn/1 -> Selector/2
  Data Store Read/1 -> Selector/1

== system ES101A_DiagcMgr/DiagcMgr/ReadNtcInfoAndDebCntr/ApplX/NonDebounced ==
  Action Port : ActionPort  ActionType=then
  CopyRight2 : Subsystem  Description=|  mask(Copyright Information){none=on}
      | Copyright info block.                                               
      |                                                                     
      | Place copyright information at the top of every subsystem in design.
      mask prompts: none "No parameters"
      mask help: Place copyright information at the top of every subsystem in design.
      mask Display:
      | NxtrConf = 'Nexteer Confidential';
      | 
      | sys = bdroot; %handle for the current model ("system")
      | first = get_param(sys,'Created');
      | first = first(end-3:end);  %year is last four digits
      | 
      | last = get_param(sys,'LastModifiedDate');
      | if isempty(last)
      |     last = datestr(now,'yyyy');
      | else
      |     last = last(end-3:end);
      | end
      | 
      | if strcmp(first,last)
      |     fprintf('%s -- Copyright %s Nexteer',NxtrConf,first)
      | else
      |     fprintf('%s -- %s%s- %s Nexteer',NxtrConf,char(169),first,last)
      | end
  Init Default Value : Constant  Value=0  OutDataTypeStr=int16
  DebCntr_ArgOut : Outport
  wires:
  Init Default Value/1 -> DebCntr_ArgOut/1

== system ES101A_DiagcMgr/DiagcMgr/ReadNtcInfoAndDebCntr/DoNothing/CopyRight2 ==

== system ES101A_DiagcMgr/DiagcMgr/ReadSnpshtData/Send out data/CopyRight2 ==

== system ES101A_DiagcMgr/DiagcMgr/RestoreNtcFltAryDft/Subsystem/CopyRight2 ==

== system ES101A_DiagcMgr/DiagcMgr/RestoreSnpshtAryDft/Subsystem/CopyRight2 ==

== system ES101A_DiagcMgr/DiagcMgr/SetNtcStsCore/Create SnapshotDataBus/CopyRight2 ==

== system ES101A_DiagcMgr/DiagcMgr/SetNtcStsCore/NtcNr is Invalid/CopyRight2 ==

== system ES101A_DiagcMgr/DiagcMgr/SetNtcStsCore/NtcNr is Valid/CopyRight2 ==

== system ES101A_DiagcMgr/DiagcMgr/SetNtcStsCore/NtcNr is Valid/Diagnostics Inhibited ==
  Action Port : ActionPort  ActionType=then
  CopyRight2 : Subsystem  Description=|  mask(Copyright Information){none=on}
      | Copyright info block.                                               
      |                                                                     
      | Place copyright information at the top of every subsystem in design.
      mask prompts: none "No parameters"
      mask help: Place copyright information at the top of every subsystem in design.
      mask Display:
      | NxtrConf = 'Nexteer Confidential';
      | 
      | sys = bdroot; %handle for the current model ("system")
      | first = get_param(sys,'Created');
      | first = first(end-3:end);  %year is last four digits
      | 
      | last = get_param(sys,'LastModifiedDate');
      | if isempty(last)
      |     last = datestr(now,'yyyy');
      | else
      |     last = last(end-3:end);
      | end
      | 
      | if strcmp(first,last)
      |     fprintf('%s -- Copyright %s Nexteer',NxtrConf,first)
      | else
      |     fprintf('%s -- %s%s- %s Nexteer',NxtrConf,char(169),first,last)
      | end
  E_OK : Constant  Value=0  OutDataTypeStr=uint8
  SetNtcSts_StdRtn : Outport
  wires:
  E_OK/1 -> SetNtcSts_StdRtn/1

== system ES101A_DiagcMgr/DiagcMgr/SetNtcStsCore/NtcNr is Valid/Diagnostics Not Inhibited ==
  NtcNr_ArgIn : Inport  OutDataTypeStr=Enum: NtcNr1
  NtcStInfo_ArgIn : Inport  Port=2
  NtcSts_ArgIn : Inport  Port=3
  DebStep_ArgIn : Inport  Port=4
  DiagcData_ArgIn : Inport  Port=5
  ProxySetNtcData_ArgIn : Inport  Port=6
  NtcInfo_ArgIn : Inport  Port=7
  NtcInfoDebCntr_ArgIn : Inport  Port=8
  SnapshotDataBus : Inport  Port=9
  Action Port : ActionPort  ActionType=else
  Compare to Zero : simulink/Logic and Bit Operations/Compare To Zero  relop=~=  OutDataTypeStr=boolean
  CopyRight2 : Subsystem  Description=|  mask(Copyright Information){none=on}
      | Copyright info block.                                               
      |                                                                     
      | Place copyright information at the top of every subsystem in design.
      mask prompts: none "No parameters"
      mask help: Place copyright information at the top of every subsystem in design.
      mask Display:
      | NxtrConf = 'Nexteer Confidential';
      | 
      | sys = bdroot; %handle for the current model ("system")
      | first = get_param(sys,'Created');
      | first = first(end-3:end);  %year is last four digits
      | 
      | last = get_param(sys,'LastModifiedDate');
      | if isempty(last)
      |     last = datestr(now,'yyyy');
      | else
      |     last = last(end-3:end);
      | end
      | 
      | if strcmp(first,last)
      |     fprintf('%s -- Copyright %s Nexteer',NxtrConf,first)
      | else
      |     fprintf('%s -- %s%s- %s Nexteer',NxtrConf,char(169),first,last)
      | end
  Data Type Conversion : DataTypeConversion  OutDataTypeStr=uint16
  FLTRESPNTCENAD_CNT_U32 : simulink/Logic and Bit Operations/Bitwise Operator  RequirementInfo={} %GIDa_593aed41_ab80_41c3_a55c_9e73ab3b96e7  logicop=AND  UseBitMask=on  BitMask=FLTRESPNTCENAD_CNT_U32  BitMaskRealWorld=Stored Integer
  Fault Response Table : Constant  Value=DiagcMgrFltResp
  If : If  IfExpression=u1 == 1
  Merge : Merge
  NtcEnabled : Subsystem  TreatAsAtomicUnit=on
  NtcNotEnabled : Subsystem  RequirementInfo={} %GIDa_04c240ca_2300_4954_9387_afe5c66cdb46  TreatAsAtomicUnit=on
  Selector : Selector  IndexMode=Zero-based  InputPortWidth=512  IndexOptions=Index vector (port)  Indices=[1 3]  OutputSizes=1
  SetNtcSts_StdRtn : Outport
  "NtcInfo_ArgOut " : Outport  Port=2
  "DiagcData_ArgOut " : Outport  Port=3
  "ProxySetNtcData_ArgOut " : Outport  Port=4
  "NtcInfoDebCntr_ArgOut " : Outport  Port=5
  wires:
  Fault Response Table/1 -> Selector/1
  Data Type Conversion/1 -> Selector/2
  NtcNr_ArgIn/1 -> NtcEnabled/1(NtcNr_ArgIn), Data Type Conversion/1
  FLTRESPNTCENAD_CNT_U32/1 -> Compare to Zero/1
  If/1 -> NtcEnabled/Action
  NtcSts_ArgIn/1 -> NtcEnabled/4(NtcSts_ArgIn)
  NtcStInfo_ArgIn/1 -> NtcEnabled/2(NtcStInfo_ArgIn)
  Selector/1 -> FLTRESPNTCENAD_CNT_U32/1
  Compare to Zero/1 -> If/1
  DebStep_ArgIn/1 -> NtcEnabled/3(DebStep_ArgIn)
  If/2 -> NtcNotEnabled/Action
  NtcNotEnabled/1(SetNtcSts_StdRtn) -> Merge/2
  NtcEnabled/5(SetNtcSts_StdRtn) -> Merge/1
  Merge/1 -> SetNtcSts_StdRtn/1
  NtcInfo_ArgIn/1 -> NtcEnabled/7(NtcInfo_ArgIn)
  DiagcData_ArgIn/1 -> NtcEnabled/5(DiagcData_ArgIn)
  ProxySetNtcData_ArgIn/1 -> NtcEnabled/6(ProxySetNtcData_ArgIn)
  NtcEnabled/1("NtcInfo_ArgOut ") -> "NtcInfo_ArgOut "/1
  NtcEnabled/3("ProxySetNtcData_ArgOut ") -> "ProxySetNtcData_ArgOut "/1
  NtcEnabled/2("DiagcData_ArgOut ") -> "DiagcData_ArgOut "/1
  NtcInfoDebCntr_ArgIn/1 -> NtcEnabled/8(NtcInfoDebCntr_ArgIn)
  NtcEnabled/4("NtcInfoDebCntr_ArgOut ") -> "NtcInfoDebCntr_ArgOut "/1
  SnapshotDataBus/1 -> NtcEnabled/9(SnapshotDataBus)

== system ES101A_DiagcMgr/DiagcMgr/SetNtcStsCore/NtcNr is Valid/Ntc Freeze Condition ==
  NtcNr : Inport
  AND : simulink/Logic and Bit Operations/Bitwise Operator  RequirementInfo={} %GIDa_35df0ee9_cca2_43c2_820c_df5695a1895c  logicop=AND  UseBitMask=off  NumInputPorts=2  BitMask=FLTRESPMFGINHBNOTINENAST_CNT_U32  BitMaskRealWorld=Stored Integer
  CopyRight2 : Subsystem  Description=|  mask(Copyright Information){none=on}
      | Copyright info block.                                               
      |                                                                     
      | Place copyright information at the top of every subsystem in design.
      mask prompts: none "No parameters"
      mask help: Place copyright information at the top of every subsystem in design.
      mask Display:
      | NxtrConf = 'Nexteer Confidential';
      | 
      | sys = bdroot; %handle for the current model ("system")
      | first = get_param(sys,'Created');
      | first = first(end-3:end);  %year is last four digits
      | 
      | last = get_param(sys,'LastModifiedDate');
      | if isempty(last)
      |     last = datestr(now,'yyyy');
      | else
      |     last = last(end-3:end);
      | end
      | 
      | if strcmp(first,last)
      |     fprintf('%s -- Copyright %s Nexteer',NxtrConf,first)
      | else
      |     fprintf('%s -- %s%s- %s Nexteer',NxtrConf,char(169),first,last)
      | end
  DTC Enable Mask : Constant  Value=DtcEnaMask
  Data Store Read : DataStoreRead  DataStoreName=DtcEnaSts
  Data Type Conversion1 : DataTypeConversion  OutDataTypeStr=uint8
  Data Type Conversion3 : DataTypeConversion  OutDataTypeStr=uint16
  FLTRESPDTCIDX_CNT_U32 : simulink/Logic and Bit Operations/Bitwise Operator  RequirementInfo={} %GIDa_344dd45f_2715_4b81_9894_441bbd7b2229  logicop=AND  UseBitMask=on  BitMask=FLTRESPDTCIDX_CNT_U32  BitMaskRealWorld=Stored Integer
  Fault Response Table1 : Constant  Value=DiagcMgrFltResp
  Selector1 : Selector  IndexMode=Zero-based  InputPortWidth=512  IndexOptions=Index vector (port)  Indices=[1 3]  OutputSizes=1
  Selector2 : Selector  IndexMode=Zero-based  InputPortWidth=512  IndexOptions=Index vector (port)  Indices=[1 3]  OutputSizes=1
  DtcEnaMask : Outport
  DTCStatus AND DTCMask : Outport  Port=2
  NtcNrRange : Outport  Port=3
  wires:
  DTC Enable Mask/1 -> Selector1/1
  Data Store Read/1 -> AND/2
  AND/1 -> DTCStatus AND DTCMask/1
  Selector1/1 -> DtcEnaMask/1, AND/1
  NtcNr/1 -> Data Type Conversion3/1
  Fault Response Table1/1 -> Selector2/1
  Data Type Conversion3/1 -> NtcNrRange/1, Selector2/2
  Selector2/1 -> FLTRESPDTCIDX_CNT_U32/1
  FLTRESPDTCIDX_CNT_U32/1 -> Data Type Conversion1/1
  Data Type Conversion1/1 -> Selector1/2

== system ES101A_DiagcMgr/DiagcMgr/UpdDtcEnaCdn/ClrBit/CopyRight2 ==

== system ES101A_DiagcMgr/DiagcMgr/UpdDtcEnaCdn/SetBit/CopyRight2 ==

== system ES101A_DiagcMgr/DiagcMgr/DiagcMgrIninCore/Initialize the NtcInfo Array/Update the ISO bits of each NTC/CopyRight2 ==

== system ES101A_DiagcMgr/DiagcMgr/DiagcMgrIninCore/Initialize the NtcInfo Array/Update the ISO bits of each NTC/Start Initialization ==
  note: NtcStInfo is not initialized to 0 explicitly in this block.
      | Since NtcStInfo is a PIM and at initialization its default value is 0, it not initialized to 0 again.
  NtcInfoIdx : Inport
  NtcInfoAry_ArgIn : Inport  Port=2
  Bus Assignment : BusAssignment  AssignedSignals=AgiCntr,Sts
  Bus Selector : BusSelector  OutputSignals=AgiCntr,Sts
  CopyRight2 : Subsystem  Description=|  mask(Copyright Information){none=on}
      | Copyright info block.                                               
      |                                                                     
      | Place copyright information at the top of every subsystem in design.
      mask prompts: none "No parameters"
      mask help: Place copyright information at the top of every subsystem in design.
      mask Display:
      | NxtrConf = 'Nexteer Confidential';
      | 
      | sys = bdroot; %handle for the current model ("system")
      | first = get_param(sys,'Created');
      | first = first(end-3:end);  %year is last four digits
      | 
      | last = get_param(sys,'LastModifiedDate');
      | if isempty(last)
      |     last = datestr(now,'yyyy');
      | else
      |     last = last(end-3:end);
      | end
      | 
      | if strcmp(first,last)
      |     fprintf('%s -- Copyright %s Nexteer',NxtrConf,first)
      | else
      |     fprintf('%s -- %s%s- %s Nexteer',NxtrConf,char(169),first,last)
      | end
  If : If  IfExpression=(u1 == 0) | (u1 > 64)
  If Action Subsystem : Subsystem  TreatAsAtomicUnit=on
  If Action Subsystem1 : Subsystem  TreatAsAtomicUnit=on
  Merge1 : Merge
  Merge2 : Merge
  Selector : Selector  IndexMode=Zero-based  InputPortWidth=22  IndexOptions=Index vector (port)  Indices=[1 3]  OutputSizes=1
  Set: DIAGCMGR_NTCINFOSTSTESTNOTCMPLTHISIGNCYC_CNT_U08 : simulink/Logic and Bit Operations/Bitwise Operator  logicop=OR  UseBitMask=on  BitMask=DIAGCMGR_NTCINFOSTSTESTNOTCMPLTHISIGNCYC_CNT_U08  BitMaskRealWorld=Stored Integer
  NtcInfoAry_ArgOut : Outport
  wires:
  Merge1/1 -> Bus Assignment/2
  If Action Subsystem/1("AgiCntr ") -> Merge1/1
  If Action Subsystem1/1(AgiCntr) -> Merge1/2
  Bus Selector/1 -> If/1, If Action Subsystem/1(AgiCntr)  "<AgiCntr>"
  Selector/1 -> Bus Assignment/1, Bus Selector/1
  Set: DIAGCMGR_NTCINFOSTSTESTNOTCMPLTHISIGNCYC_CNT_U08/1 -> Bus Assignment/3
  Merge2/1 -> Set: DIAGCMGR_NTCINFOSTSTESTNOTCMPLTHISIGNCYC_CNT_U08/1
  NtcInfoIdx/1 -> Selector/2
  Bus Selector/2 -> If Action Subsystem1/1(Sts), If Action Subsystem/2(Sts)  "<Sts>"
  If Action Subsystem/2("Sts ") -> Merge2/1
  If Action Subsystem1/2("Sts ") -> Merge2/2
  Bus Assignment/1 -> NtcInfoAry_ArgOut/1
  NtcInfoAry_ArgIn/1 -> Selector/1
  If/1 -> If Action Subsystem1/Action
  If/2 -> If Action Subsystem/Action

== system ES101A_DiagcMgr/DiagcMgr/DiagcMgrIninCore/Update DiagcSts and DiagcMgrActv/Dual Inverter/CopyRight2 ==

== system ES101A_DiagcMgr/DiagcMgr/DiagcMgrIninCore/Update DiagcSts and DiagcMgrActv/Single Inverter/CopyRight2 ==

== system ES101A_DiagcMgr/DiagcMgr/DiagcMgrIninCore/Update NtcInfoAry From NvM/Update NtcInfoAry/CopyRight2 ==

== system ES101A_DiagcMgr/DiagcMgr/DiagcMgrIninCore/Update NtcInfoAry From NvM/Update NtcInfoAry/Update NtcInfoAry Aging Counter And Confirmed Bit ==
  NtcFltIdx : Inport
  AppIdx_ArgIn : Inport  Port=2
  NtcInfoAry_ArgIn : Inport  Port=3
  Bus Selector1 : BusSelector  OutputSignals=NtcNr,AgiCntr,Sts
  CopyRight2 : Subsystem  Description=|  mask(Copyright Information){none=on}
      | Copyright info block.                                               
      |                                                                     
      | Place copyright information at the top of every subsystem in design.
      mask prompts: none "No parameters"
      mask help: Place copyright information at the top of every subsystem in design.
      mask Display:
      | NxtrConf = 'Nexteer Confidential';
      | 
      | sys = bdroot; %handle for the current model ("system")
      | first = get_param(sys,'Created');
      | first = first(end-3:end);  %year is last four digits
      | 
      | last = get_param(sys,'LastModifiedDate');
      | if isempty(last)
      |     last = datestr(now,'yyyy');
      | else
      |     last = last(end-3:end);
      | end
      | 
      | if strcmp(first,last)
      |     fprintf('%s -- Copyright %s Nexteer',NxtrConf,first)
      | else
      |     fprintf('%s -- %s%s- %s Nexteer',NxtrConf,char(169),first,last)
      | end
  Data Store Read1 : DataStoreRead  DataStoreName=DiagcMgrNtcFltAry  DataStoreElements=DiagcMgrNtcFltAry(:)
  Data Type Conversion : DataTypeConversion  OutDataTypeStr=uint16
  If Action : Subsystem
  If1 : If  IfExpression=(u1 > 0)&(u1 < 512)  ShowElse=off
  Selector1 : Selector  IndexMode=Zero-based  InputPortWidth=20  IndexOptions=Index vector (port)  Indices=[1 3]  OutputSizes=1
  NtcInfoAry_ArgOut : Outport
  wires:
  NtcFltIdx/1 -> Selector1/2
  Bus Selector1/1 -> If Action/1(NtcNr), Data Type Conversion/1  "<NtcNr>"
  Selector1/1 -> Bus Selector1/1
  Data Store Read1/1 -> Selector1/1
  AppIdx_ArgIn/1 -> If Action/4(ApplIdx)
  Data Type Conversion/1 -> If1/1
  If1/1 -> If Action/Action
  Bus Selector1/3 -> If Action/3(Sts)  "<Sts>"
  Bus Selector1/2 -> If Action/2(AgiCntr_ArgIn)  "<AgiCntr>"
  NtcInfoAry_ArgIn/1 -> If Action/5(NtcInfoAry_ArgIn)
  If Action/1(NtcInfoAry_ArgOut) -> NtcInfoAry_ArgOut/1

== system ES101A_DiagcMgr/DiagcMgr/DiagcMgrPer1/Update OutpDiagcData/GetDiagcDataApplX/CopyRight2 ==

== system ES101A_DiagcMgr/DiagcMgr/DiagcMgrPer1/Update the Reduced Performance Outputs/FltInj_logl/CopyRight1 ==

== system ES101A_DiagcMgr/DiagcMgr/DiagcMgrPer1/Update the Reduced Performance Outputs/FltInj_logl1/CopyRight1 ==

== system ES101A_DiagcMgr/DiagcMgr/DiagcMgrPer2/Clear All DTCs/Call DEM & Update DtcIdxPrevSts/CopyRight2 ==
